simulink model "PD2"  (R2015a)
settings: Solver=ode1  SolverMode=SingleTasking  StartTime=0.0  StopTime=inf  FixedStep=0.005  RelTol=1e-3
values from neighbouring files (symbols this model uses):
  K = lqr(A,B,Q,R,N)    [LM1SLQR.m]
libraries: gtbox x6
settings Model: SimulationMode=external  ExtModeTrigDuration=200000  Creator=Administrator  LastModifiedBy=elec3200
settings DataIOCC: SignalLoggingSaveFormat=ModelDataLogs  SignalLoggingName=sigsOut
settings OptimizationCC: ExpressionDepthLimit=2147483647  InitFltsAndDblsToZero=on
settings DebuggingCC: SaveWithParameterizedLinksMsg=none  UnderspecifiedInitializationDetection=Classic  MergeDetectMultiDrivingBlocksExec=none  SignalResolutionControl=TryResolveAllWithWarning  MultiTaskDSMMsg=warning  MultiTaskCondExecSysMsg=none  FcnCallInpInsideContextMsg=UseLocalSettings  StateNameClashWarn=warning
settings HardwareCC: ProdBitPerLong=64  ProdBitPerPointer=64  ProdIntDivRoundTo=Zero  ProdEndianess=LittleEndian  ProdWordSize=64  ProdHWDeviceType=Intel->x86-64  TargetBitPerLong=64  TargetBitPerPointer=64  TargetIntDivRoundTo=Zero  TargetEndianess=LittleEndian  TargetWordSize=64  TargetHWDeviceType=Intel->x86-64
settings RTWCC: SystemTargetFile=rtwin.tlc  TemplateMakefile=rtwin.tmf  Description=Real-Time Windows Target
settings RTWinTargetCC: TargetFcnLib=ansi_tfl_tmw.mat  TargetPreCompLibLocation=C:\Program Files\MATLAB\R2015a\toolbox\sldrt\lib\win64  ModelReferenceCompliant=off  CompOptLevelCompliant=off

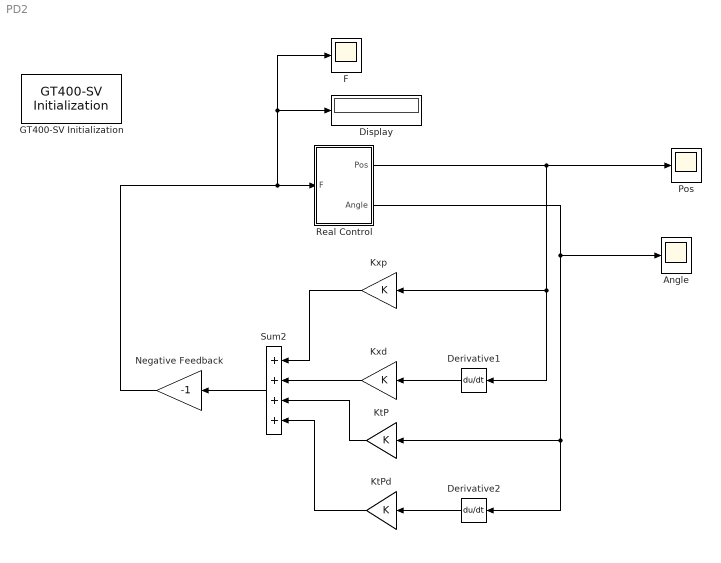
== system PD2 ==
  Angle : Scope
      settings: TickLabels=on  TimeRange=200  YMin=-3.5  YMax=3.5  SaveName=Angle  MaxDataPoints=10000
  Derivative1 : Derivative
  Derivative2 : Derivative
  Display : Display
  "F " : Scope
      settings: TickLabels=on  TimeRange=200  YMin=-17.5  YMax=20  SaveName=Pos1  MaxDataPoints=10000
  GT400-SV Initialization : gtbox/GT-400-SV Function Blocks/GT400-SV Initialization  Priority=0  openloop=1  comport=0
  KtP : Gain  Gain=K
  KtPd : Gain  Gain=K
  Kxd : Gain  Gain=K
  Kxp : Gain  Gain=K
  Negative Feedback : Gain  Gain=-1
  Pos : Scope
      settings: TickLabels=on  TimeRange=200  YMin=-0.2  YMax=0.125  SaveName=Pos  MaxDataPoints=10000
  Real Control : Subsystem
  Sum2 : Sum  Inputs=++++
  wires:
  Negative Feedback/1 -> Display/1, "F "/1, Real Control/1(F)
  Sum2/1 -> Negative Feedback/1
  Kxp/1 -> Sum2/1
  Kxd/1 -> Sum2/2
  Derivative1/1 -> Kxd/1
  Real Control/1(Pos) -> Kxp/1, Derivative1/1, Pos/1
  KtP/1 -> Sum2/3
  KtPd/1 -> Sum2/4
  Derivative2/1 -> KtPd/1
  Real Control/2(Angle) -> Angle/1, Derivative2/1, KtP/1

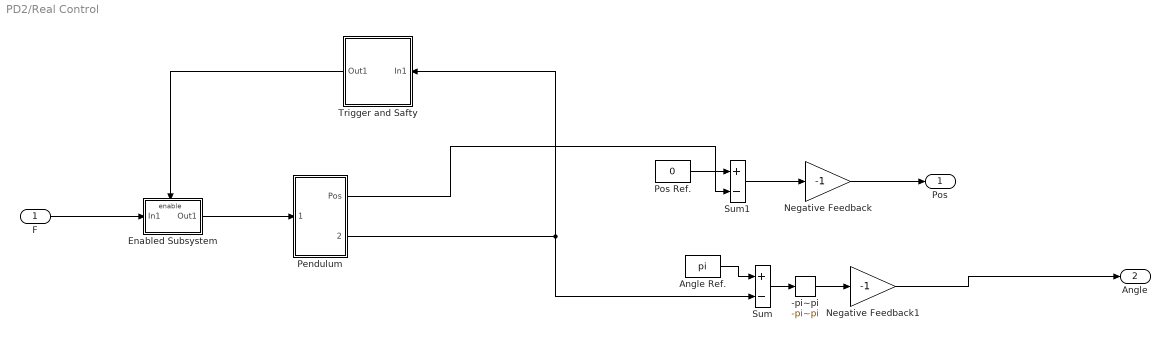
== system PD2/Real Control ==
  F : Inport
  " -pi~pi" : gtbox/GT-400-SV Function Blocks/ -pi~pi
  Angle Ref. : Constant  Value=pi
  Enabled Subsystem : Subsystem  TreatAsAtomicUnit=on
  Negative Feedback : Gain  Gain=-1
  Negative Feedback1 : Gain  Gain=-1
  Pendulum : Subsystem
  Pos Ref. : Constant  Value=0
  Sum : Sum  Inputs=+-  SaturateOnIntegerOverflow=on
  Sum1 : Sum  Inputs=+-  SaturateOnIntegerOverflow=on
  Trigger and Safty : Subsystem
  Pos : Outport
  Angle : Outport  Port=2
  wires:
  F/1 -> Enabled Subsystem/1(In1)
  Enabled Subsystem/1(Out1) -> Pendulum/1(Cmd)
  Trigger and Safty/1(Out1) -> Enabled Subsystem/Enable
  Pendulum/2(Angle) -> Sum/2, Trigger and Safty/1(In1)
  Pos Ref./1 -> Sum1/1
  Pendulum/1(Pos) -> Sum1/2
  Sum1/1 -> Negative Feedback/1
  Angle Ref./1 -> Sum/1
  Sum/1 -> " -pi~pi"/1
  " -pi~pi"/1 -> Negative Feedback1/1
  Negative Feedback/1 -> Pos/1
  Negative Feedback1/1 -> Angle/1

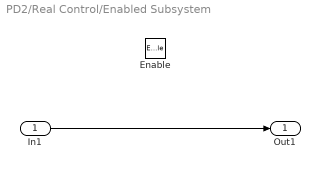
== system PD2/Real Control/Enabled Subsystem ==
  In1 : Inport
  Enable : EnablePort
  Out1 : Outport
  wires:
  In1/1 -> Out1/1

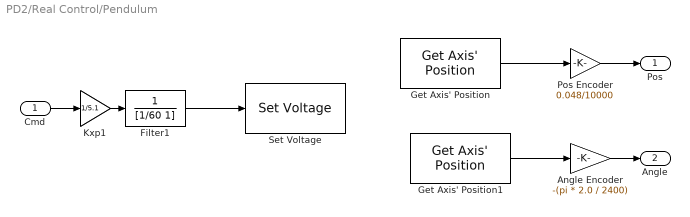
== system PD2/Real Control/Pendulum ==
  Cmd : Inport
  Angle Encoder : Gain  Gain=-(pi * 2.0 / 2400)  SaturateOnIntegerOverflow=on  OutDataTypeStr=Inherit: Same as input  ParamDataTypeStr=Inherit: Same as input
  Filter1 : TransferFcn  Denominator=[1/60 1]
  Get Axis' Position : gtbox/GT-400-SV Function Blocks/Get Axis' Position  Priority=1  axis=1
  Get Axis' Position1 : gtbox/GT-400-SV Function Blocks/Get Axis' Position  Priority=1  axis=2
  Kxp1 : Gain  Gain=1/5.1
  Pos Encoder : Gain  Gain=0.048/10000  SaturateOnIntegerOverflow=on  OutDataTypeStr=Inherit: Same as input  ParamDataTypeStr=Inherit: Same as input
  Set Voltage : gtbox/GT-400-SV Function Blocks/Set Voltage  Priority=1  axis=1  back_cmd=1  back_pos=20000
  Pos : Outport
  Angle : Outport  Port=2
  wires:
  Angle Encoder/1 -> Angle/1
  Pos Encoder/1 -> Pos/1
  Get Axis' Position/1 -> Pos Encoder/1
  Get Axis' Position1/1 -> Angle Encoder/1
  Cmd/1 -> Kxp1/1
  Kxp1/1 -> Filter1/1
  Filter1/1 -> Set Voltage/1

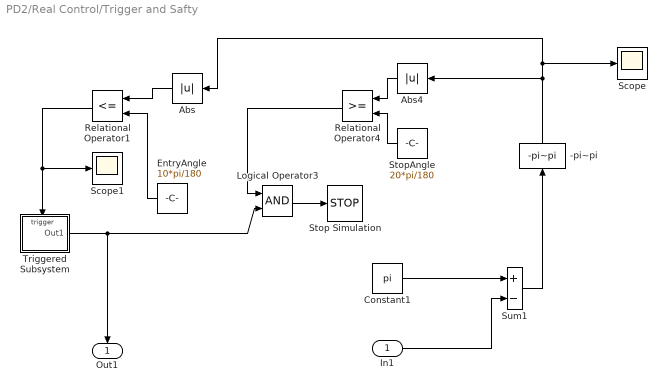
== system PD2/Real Control/Trigger and Safty ==
  In1 : Inport
  " -pi~pi" : gtbox/GT-400-SV Function Blocks/ -pi~pi
  Abs : Abs  SaturateOnIntegerOverflow=on
  Abs4 : Abs  SaturateOnIntegerOverflow=on
  Constant1 : Constant  Value=pi
  EntryAngle : Constant  Value=10*pi/180
  Logical Operator3 : Logic  AllPortsSameDT=off
  Relational Operator1 : RelationalOperator  Operator=<=
  Relational Operator4 : RelationalOperator
  Scope : Scope
      settings: YMin=-3.134  YMax=-3.123
  Scope1 : Scope
      settings: YMin=-3.134  YMax=-3.123
  Stop Simulation : Stop
  StopAngle : Constant  Value=20*pi/180
  Sum1 : Sum  Inputs=+-  SaturateOnIntegerOverflow=on
  Triggered Subsystem : Subsystem  TreatAsAtomicUnit=on
  Out1 : Outport
  wires:
  Relational Operator4/1 -> Logical Operator3/1
  StopAngle/1 -> Relational Operator4/2
  Abs4/1 -> Relational Operator4/1
  Abs/1 -> Relational Operator1/1
  EntryAngle/1 -> Relational Operator1/2
  Relational Operator1/1 -> Scope1/1, Triggered Subsystem/Trigger
  Triggered Subsystem/1(Out1) -> Logical Operator3/2, Out1/1
  Logical Operator3/1 -> Stop Simulation/1
  " -pi~pi"/1 -> Abs4/1, Scope/1, Abs/1
  Constant1/1 -> Sum1/1
  In1/1 -> Sum1/2
  Sum1/1 -> " -pi~pi"/1

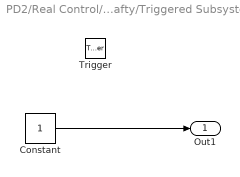
== system PD2/Real Control/Trigger and Safty/Triggered Subsystem ==
  Trigger : TriggerPort
  Constant : Constant
  Out1 : Outport  InitialOutput=0
  wires:
  Constant/1 -> Out1/1
